simulink model "Model_Te02_R2020b"  (R2022b)
settings: Solver=FixedStepAuto  StartTime=0.0  StopTime=25  FixedStep=0.2  RelTol=1e-3
undefined symbols (not defined in the file or in its folder): serial
libraries: instrumentseriallib x3
settings Model: Creator=berci  LastModifiedBy=rus_d
settings SolverCC: AlgebraicLoopSolver=TrustRegion
settings DataIOCC: ReturnWorkspaceOutputs=off
settings DebuggingCC: UnconnectedInputMsg=warning  UnconnectedOutputMsg=warning  UnconnectedLineMsg=warning  SFMachineParentedDataDiag=warning  ArithmeticOperatorsInVariantConditions=warning
settings ModelReferenceCC: EnableRefExpFcnMdlSchedulingChecks=on
settings SFSimCC: SimUseLocalCustomCode=off  CustomCodeUndefinedFunction=UseInterfaceOnly
settings RTWCC: RTWUseLocalCustomCode=off  DLArmComputeVersion=19.05

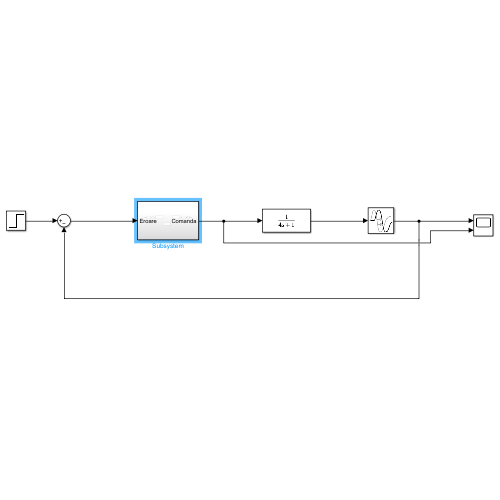
[thumbnail: Simulink's stored preview of the top-level diagram]
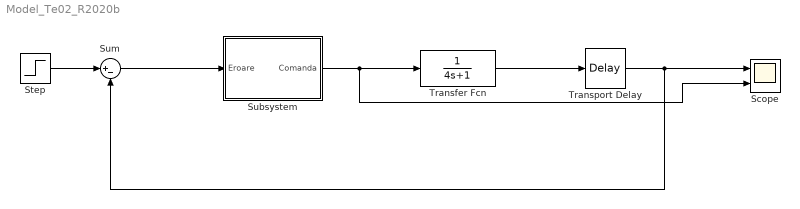
== system Model_Te02_R2020b ==
  Scope : Scope  NumInputPorts=2
  Step : Step  Time=0  SampleTime=0.4
  Subsystem : Subsystem
  Sum : Sum  Inputs=|+-
  Transfer Fcn : TransferFcn  Numerator=1  Denominator=[4 1]
  Transport Delay : TransportDelay  DelayTime=2
  wires:
  Transport Delay/1 -> Sum/2, Scope/1
  Transfer Fcn/1 -> Transport Delay/1
  Subsystem/1(Comanda) -> Scope/2, Transfer Fcn/1
  Sum/1 -> Subsystem/1(Eroare)
  Step/1 -> Sum/1

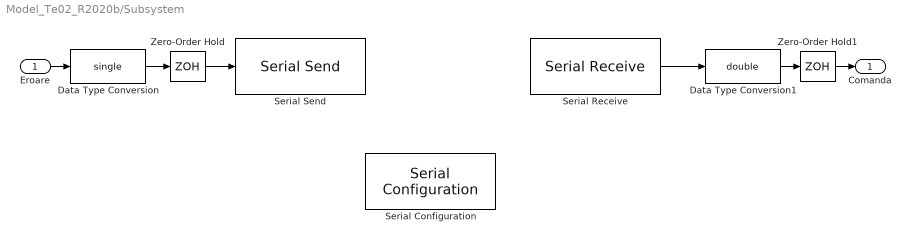
== system Model_Te02_R2020b/Subsystem ==
  Eroare : Inport
  Data Type Conversion : DataTypeConversion  OutDataTypeStr=single  SaturateOnIntegerOverflow=off  RndMeth=Floor
  Data Type Conversion1 : DataTypeConversion  OutDataTypeStr=double  SaturateOnIntegerOverflow=off  RndMeth=Floor
  Serial Configuration : instrumentseriallib/Serial Configuration  Priority=-200000  PortSel=COM3  Port=COM3  ComPort=COM3  BaudRate=9600  DataBits=8  Parity=none  StopBits=1  ByteOrder=little-endian  FlowControl=none  Timeout=10  SimulateUsing=Interpreted execution  BlockInModel=on  aMode=1
  Serial Receive : instrumentseriallib/Serial Receive  PortSel=COM3  Port=COM3  ComPort=COM3  ObjConstructor=serial('COM3');  DataType=single  SaveDataType=uint8  ToggleHeader=off  Header=[]  ToggleTerminator=off  Terminator=<none>  CustomTerminator=[]  InputFormat=Column major  ToggleDataSize=on  DataSize=[1 1]  EnableBlockingMode=on  ActionDataUnavailable=Output last received value  ActionWhenDataUnavailable=Output last received value  CustomValue=0  SampleTime=0.4  SimulateUsing=Interpreted execution  BlockInModel=on  aMode=1
  Serial Send : instrumentseriallib/Serial Send  PortSel=COM3  Port=COM3  ComPort=COM3  Header=[]  Terminator=<none>  CustomTerminator=[]  EnableBlockingMode=on  SimulateUsing=Interpreted execution  BlockInModel=on  aMode=1
  Zero-Order Hold : ZeroOrderHold  SampleTime=0.4
  Zero-Order Hold1 : ZeroOrderHold  SampleTime=0.2
  Comanda : Outport  VectorParamsAs1DForOutWhenUnconnected=off
  wires:
  Eroare/1 -> Data Type Conversion/1
  Zero-Order Hold1/1 -> Comanda/1
  Data Type Conversion1/1 -> Zero-Order Hold1/1
  Serial Receive/1 -> Data Type Conversion1/1
  Zero-Order Hold/1 -> Serial Send/1
  Data Type Conversion/1 -> Zero-Order Hold/1
